simulink model "Microgrid_W"  (R2020a)
settings: Solver=ode15s  StartTime=0  StopTime=1440*1  MaxStep=1  RelTol=1e-3
libraries: simulink x4214, powerlib x685, simulink_extras x28, Microgrid_Library x18, powerlib_meascontrol x12
(part 44 of 48)

== system Microgrid_W/House 5 W2/Tv/D1 ==
  Add : Sum
  Clock : Clock
  Constant : Constant
  Constant1 : Constant  Value=0
  Gain : Gain  Gain=t
  Interval Test : simulink/Logic and Bit Operations/Interval Test  IntervalClosedRight=on  uplimit=TV_Off_1  IntervalClosedLeft=on  lowlimit=TV_On_1  OutDataTypeStr=boolean
  Interval Test1 : simulink/Logic and Bit Operations/Interval Test  IntervalClosedRight=on  uplimit=TV_Off_2  IntervalClosedLeft=on  lowlimit=TV_On_2  OutDataTypeStr=boolean
  Switch : Switch  Criteria=u2 > Threshold  Threshold=0.5
  Switch1 : Switch  Criteria=u2 > Threshold  Threshold=0.5
  Out1 : Outport  VectorParamsAs1DForOutWhenUnconnected=off
  wires:
  Clock/1 -> Gain/1
  Interval Test/1 -> Switch/2
  Switch/1 -> Add/1
  Interval Test1/1 -> Switch1/2
  Add/1 -> Out1/1
  Constant1/1 -> Switch/3, Switch1/3
  Constant/1 -> Switch/1, Switch1/1
  Switch1/1 -> Add/2
  Gain/1 -> Interval Test1/1, Interval Test/1

== system Microgrid_W/House 5 W2/Tv/D2 ==
  Add : Sum
  Clock : Clock
  Constant : Constant
  Constant1 : Constant  Value=0
  Gain : Gain  Gain=t
  Interval Test : simulink/Logic and Bit Operations/Interval Test  IntervalClosedRight=on  uplimit=TV_Off_1+86400  IntervalClosedLeft=on  lowlimit=TV_On_1+86400  OutDataTypeStr=boolean
  Interval Test1 : simulink/Logic and Bit Operations/Interval Test  IntervalClosedRight=on  uplimit=TV_Off_2+86400  IntervalClosedLeft=on  lowlimit=TV_On_2+86400  OutDataTypeStr=boolean
  Switch : Switch  Criteria=u2 > Threshold  Threshold=0.5
  Switch1 : Switch  Criteria=u2 > Threshold  Threshold=0.5
  Out1 : Outport  VectorParamsAs1DForOutWhenUnconnected=off
  wires:
  Clock/1 -> Gain/1
  Gain/1 -> Interval Test/1, Interval Test1/1
  Switch1/1 -> Add/2
  Constant/1 -> Switch1/1, Switch/1
  Constant1/1 -> Switch1/3, Switch/3
  Add/1 -> Out1/1
  Interval Test1/1 -> Switch1/2
  Switch/1 -> Add/1
  Interval Test/1 -> Switch/2

== system Microgrid_W/House 5 W2/Tv/D3 ==
  Add : Sum
  Clock : Clock
  Constant : Constant
  Constant1 : Constant  Value=0
  Gain : Gain  Gain=t
  Interval Test : simulink/Logic and Bit Operations/Interval Test  IntervalClosedRight=on  uplimit=TV_Off_1+86400*2  IntervalClosedLeft=on  lowlimit=TV_On_1+86400*2  OutDataTypeStr=boolean
  Interval Test1 : simulink/Logic and Bit Operations/Interval Test  IntervalClosedRight=on  uplimit=TV_Off_2+86400*2  IntervalClosedLeft=on  lowlimit=TV_On_2+86400*2  OutDataTypeStr=boolean
  Switch : Switch  Criteria=u2 > Threshold  Threshold=0.5
  Switch1 : Switch  Criteria=u2 > Threshold  Threshold=0.5
  Out1 : Outport  VectorParamsAs1DForOutWhenUnconnected=off
  wires:
  Clock/1 -> Gain/1
  Interval Test/1 -> Switch/2
  Switch/1 -> Add/1
  Interval Test1/1 -> Switch1/2
  Add/1 -> Out1/1
  Constant1/1 -> Switch/3, Switch1/3
  Constant/1 -> Switch/1, Switch1/1
  Switch1/1 -> Add/2
  Gain/1 -> Interval Test1/1, Interval Test/1

== system Microgrid_W/House 5 W2/Tv/D4 ==
  Add : Sum
  Clock : Clock
  Constant : Constant
  Constant1 : Constant  Value=0
  Gain : Gain  Gain=t
  Interval Test : simulink/Logic and Bit Operations/Interval Test  IntervalClosedRight=on  uplimit=TV_Off_1+86400*3  IntervalClosedLeft=on  lowlimit=TV_On_1+86400*3  OutDataTypeStr=boolean
  Interval Test1 : simulink/Logic and Bit Operations/Interval Test  IntervalClosedRight=on  uplimit=TV_Off_2+86400*3  IntervalClosedLeft=on  lowlimit=TV_On_2+86400*3  OutDataTypeStr=boolean
  Switch : Switch  Criteria=u2 > Threshold  Threshold=0.5
  Switch1 : Switch  Criteria=u2 > Threshold  Threshold=0.5
  Out1 : Outport  VectorParamsAs1DForOutWhenUnconnected=off
  wires:
  Clock/1 -> Gain/1
  Gain/1 -> Interval Test/1, Interval Test1/1
  Switch1/1 -> Add/2
  Constant/1 -> Switch1/1, Switch/1
  Constant1/1 -> Switch1/3, Switch/3
  Add/1 -> Out1/1
  Interval Test1/1 -> Switch1/2
  Switch/1 -> Add/1
  Interval Test/1 -> Switch/2

== system Microgrid_W/House 5 W2/Tv/D5 ==
  Add : Sum
  Clock : Clock
  Constant : Constant
  Constant1 : Constant  Value=0
  Gain : Gain  Gain=t
  Interval Test : simulink/Logic and Bit Operations/Interval Test  IntervalClosedRight=on  uplimit=TV_Off_1+86400*4  IntervalClosedLeft=on  lowlimit=TV_On_1+86400*4  OutDataTypeStr=boolean
  Interval Test1 : simulink/Logic and Bit Operations/Interval Test  IntervalClosedRight=on  uplimit=TV_Off_2+86400*4  IntervalClosedLeft=on  lowlimit=TV_On_2+86400*4  OutDataTypeStr=boolean
  Switch : Switch  Criteria=u2 > Threshold  Threshold=0.5
  Switch1 : Switch  Criteria=u2 > Threshold  Threshold=0.5
  Out1 : Outport  VectorParamsAs1DForOutWhenUnconnected=off
  wires:
  Clock/1 -> Gain/1
  Interval Test/1 -> Switch/2
  Switch/1 -> Add/1
  Interval Test1/1 -> Switch1/2
  Add/1 -> Out1/1
  Constant1/1 -> Switch/3, Switch1/3
  Constant/1 -> Switch/1, Switch1/1
  Switch1/1 -> Add/2
  Gain/1 -> Interval Test1/1, Interval Test/1

== system Microgrid_W/House 5 W2/Tv/D6 ==
  Add : Sum
  Clock : Clock
  Constant : Constant
  Constant1 : Constant  Value=0
  Gain : Gain  Gain=t
  Interval Test : simulink/Logic and Bit Operations/Interval Test  IntervalClosedRight=on  uplimit=TV_Off_1+86400*5  IntervalClosedLeft=on  lowlimit=TV_On_1+86400*5  OutDataTypeStr=boolean
  Interval Test1 : simulink/Logic and Bit Operations/Interval Test  IntervalClosedRight=on  uplimit=TV_Off_2+86400*5  IntervalClosedLeft=on  lowlimit=TV_On_2+86400*5  OutDataTypeStr=boolean
  Switch : Switch  Criteria=u2 > Threshold  Threshold=0.5
  Switch1 : Switch  Criteria=u2 > Threshold  Threshold=0.5
  Out1 : Outport  VectorParamsAs1DForOutWhenUnconnected=off
  wires:
  Clock/1 -> Gain/1
  Gain/1 -> Interval Test/1, Interval Test1/1
  Switch1/1 -> Add/2
  Constant/1 -> Switch1/1, Switch/1
  Constant1/1 -> Switch1/3, Switch/3
  Add/1 -> Out1/1
  Interval Test1/1 -> Switch1/2
  Switch/1 -> Add/1
  Interval Test/1 -> Switch/2

== system Microgrid_W/House 5 W2/Tv/D7 ==
  Add : Sum
  Clock : Clock
  Constant : Constant
  Constant1 : Constant  Value=0
  Gain : Gain  Gain=t
  Interval Test : simulink/Logic and Bit Operations/Interval Test  IntervalClosedRight=on  uplimit=TV_Off_1+86400*6  IntervalClosedLeft=on  lowlimit=TV_On_1+86400*6  OutDataTypeStr=boolean
  Interval Test1 : simulink/Logic and Bit Operations/Interval Test  IntervalClosedRight=on  uplimit=TV_Off_2+86400*6  IntervalClosedLeft=on  lowlimit=TV_On_2+86400*6  OutDataTypeStr=boolean
  Switch : Switch  Criteria=u2 > Threshold  Threshold=0.5
  Switch1 : Switch  Criteria=u2 > Threshold  Threshold=0.5
  Out1 : Outport  VectorParamsAs1DForOutWhenUnconnected=off
  wires:
  Clock/1 -> Gain/1
  Interval Test/1 -> Switch/2
  Switch/1 -> Add/1
  Interval Test1/1 -> Switch1/2
  Add/1 -> Out1/1
  Constant1/1 -> Switch/3, Switch1/3
  Constant/1 -> Switch/1, Switch1/1
  Switch1/1 -> Add/2
  Gain/1 -> Interval Test1/1, Interval Test/1

== system Microgrid_W/House 5 W2/Water tank/Thermostat ==
  In1 : Inport
  Compare To Constant : simulink/Logic and Bit Operations/Compare To Constant  relop=>=  const=T_High_WH  OutDataTypeStr=boolean
  Compare To Constant1 : simulink/Logic and Bit Operations/Compare To Constant  relop=<=  const=T_Low_WH  OutDataTypeStr=boolean
  Constant : Constant  Value=0
  Constant1 : Constant
  S-R Flip-Flop : simulink_extras/Flip Flops/S-R Flip-Flop  initial_condition=0
  Switch : Switch  Criteria=u2 > Threshold  Threshold=0.5
  Out1 : Outport  VectorParamsAs1DForOutWhenUnconnected=off
  wires:
  Constant/1 -> Switch/3
  Constant1/1 -> Switch/1
  Switch/1 -> Out1/1
  S-R Flip-Flop/1 -> Switch/2
  Compare To Constant1/1 -> S-R Flip-Flop/1
  Compare To Constant/1 -> S-R Flip-Flop/2
  In1/1 -> Compare To Constant/1, Compare To Constant1/1

== system Microgrid_W/House 5 W3/Heater/D1 ==
  Clock : Clock
  Constant : Constant
  Constant1 : Constant  Value=0
  Gain : Gain  Gain=t
  Interval Test : simulink/Logic and Bit Operations/Interval Test  IntervalClosedRight=on  uplimit=Heater_Off_1  IntervalClosedLeft=on  lowlimit=Heater_On_1  OutDataTypeStr=boolean
  Switch : Switch  Criteria=u2 > Threshold  Threshold=0.5
  Out1 : Outport  VectorParamsAs1DForOutWhenUnconnected=off
  wires:
  Interval Test/1 -> Switch/2
  Switch/1 -> Out1/1
  Constant1/1 -> Switch/3
  Constant/1 -> Switch/1
  Gain/1 -> Interval Test/1
  Clock/1 -> Gain/1

== system Microgrid_W/House 5 W3/Heater/D2 ==
  Clock : Clock
  Constant : Constant
  Constant1 : Constant  Value=0
  Gain : Gain  Gain=t
  Interval Test : simulink/Logic and Bit Operations/Interval Test  IntervalClosedRight=on  uplimit=Heater_Off_1+86400  IntervalClosedLeft=on  lowlimit=Heater_On_1+86400  OutDataTypeStr=boolean
  Switch : Switch  Criteria=u2 > Threshold  Threshold=0.5
  Out1 : Outport  VectorParamsAs1DForOutWhenUnconnected=off
  wires:
  Constant/1 -> Switch/1
  Constant1/1 -> Switch/3
  Switch/1 -> Out1/1
  Interval Test/1 -> Switch/2
  Gain/1 -> Interval Test/1
  Clock/1 -> Gain/1

== system Microgrid_W/House 5 W3/Heater/D3 ==
  Clock : Clock
  Constant : Constant
  Constant1 : Constant  Value=0
  Gain : Gain  Gain=t
  Interval Test : simulink/Logic and Bit Operations/Interval Test  IntervalClosedRight=on  uplimit=Heater_Off_1+86400*2  IntervalClosedLeft=on  lowlimit=Heater_On_1+86400*2  OutDataTypeStr=boolean
  Switch : Switch  Criteria=u2 > Threshold  Threshold=0.5
  Out1 : Outport  VectorParamsAs1DForOutWhenUnconnected=off
  wires:
  Interval Test/1 -> Switch/2
  Switch/1 -> Out1/1
  Constant1/1 -> Switch/3
  Constant/1 -> Switch/1
  Gain/1 -> Interval Test/1
  Clock/1 -> Gain/1

== system Microgrid_W/House 5 W3/Heater/D4 ==
  Clock : Clock
  Constant : Constant
  Constant1 : Constant  Value=0
  Gain : Gain  Gain=t
  Interval Test : simulink/Logic and Bit Operations/Interval Test  IntervalClosedRight=on  uplimit=Heater_Off_1+86400*3  IntervalClosedLeft=on  lowlimit=Heater_On_1+86400*3  OutDataTypeStr=boolean
  Switch : Switch  Criteria=u2 > Threshold  Threshold=0.5
  Out1 : Outport  VectorParamsAs1DForOutWhenUnconnected=off
  wires:
  Constant/1 -> Switch/1
  Constant1/1 -> Switch/3
  Switch/1 -> Out1/1
  Interval Test/1 -> Switch/2
  Gain/1 -> Interval Test/1
  Clock/1 -> Gain/1

== system Microgrid_W/House 5 W3/Heater/D5 ==
  Clock : Clock
  Constant : Constant
  Constant1 : Constant  Value=0
  Gain : Gain  Gain=t
  Interval Test : simulink/Logic and Bit Operations/Interval Test  IntervalClosedRight=on  uplimit=Heater_Off_1+86400*4  IntervalClosedLeft=on  lowlimit=Heater_On_1+86400*4  OutDataTypeStr=boolean
  Switch : Switch  Criteria=u2 > Threshold  Threshold=0.5
  Out1 : Outport  VectorParamsAs1DForOutWhenUnconnected=off
  wires:
  Interval Test/1 -> Switch/2
  Switch/1 -> Out1/1
  Constant1/1 -> Switch/3
  Constant/1 -> Switch/1
  Gain/1 -> Interval Test/1
  Clock/1 -> Gain/1

== system Microgrid_W/House 5 W3/Heater/D6 ==
  Clock : Clock
  Constant : Constant
  Constant1 : Constant  Value=0
  Gain : Gain  Gain=t
  Interval Test : simulink/Logic and Bit Operations/Interval Test  IntervalClosedRight=on  uplimit=Heater_Off_1+86400*5  IntervalClosedLeft=on  lowlimit=Heater_On_1+86400*5  OutDataTypeStr=boolean
  Switch : Switch  Criteria=u2 > Threshold  Threshold=0.5
  Out1 : Outport  VectorParamsAs1DForOutWhenUnconnected=off
  wires:
  Gain/1 -> Interval Test/1
  Constant/1 -> Switch/1
  Constant1/1 -> Switch/3
  Switch/1 -> Out1/1
  Interval Test/1 -> Switch/2
  Clock/1 -> Gain/1

== system Microgrid_W/House 5 W3/Heater/D7 ==
  Clock : Clock
  Constant : Constant
  Constant1 : Constant  Value=0
  Gain : Gain  Gain=t
  Interval Test : simulink/Logic and Bit Operations/Interval Test  IntervalClosedRight=on  uplimit=Heater_Off_1+86400*6  IntervalClosedLeft=on  lowlimit=Heater_On_1+86400*6  OutDataTypeStr=boolean
  Switch : Switch  Criteria=u2 > Threshold  Threshold=0.5
  Out1 : Outport  VectorParamsAs1DForOutWhenUnconnected=off
  wires:
  Interval Test/1 -> Switch/2
  Switch/1 -> Out1/1
  Constant1/1 -> Switch/3
  Constant/1 -> Switch/1
  Gain/1 -> Interval Test/1
  Clock/1 -> Gain/1

== system Microgrid_W/House 5 W3/Kettle/D1 ==
  Add : Sum  Inputs=+++
  Clock : Clock
  Compare To Zero : simulink/Logic and Bit Operations/Compare To Zero  relop=>  OutDataTypeStr=boolean
  Compare To Zero1 : simulink/Logic and Bit Operations/Compare To Zero  relop=>  OutDataTypeStr=boolean
  Compare To Zero2 : simulink/Logic and Bit Operations/Compare To Zero  relop=>  OutDataTypeStr=boolean
  Constant : Constant
  Constant{1..2,5,8} (4 alike) : Constant  Value=0
  Constant3 : Constant  Value=Jug_On_1
  Constant4 : Constant
  Constant6 : Constant  Value=Jug_On_2
  Constant7 : Constant
  Constant9 : Constant  Value=Jug_On_3
  Gain : Gain  Gain=t
  Interval Test : simulink/Logic and Bit Operations/Interval Test  IntervalClosedRight=on  uplimit=Jug_On_1+180  IntervalClosedLeft=on  lowlimit=Jug_On_1  OutDataTypeStr=boolean
  Interval Test1 : simulink/Logic and Bit Operations/Interval Test  IntervalClosedRight=on  uplimit=Jug_On_2+180  IntervalClosedLeft=on  lowlimit=Jug_On_2  OutDataTypeStr=boolean
  Interval Test2 : simulink/Logic and Bit Operations/Interval Test  IntervalClosedRight=on  uplimit=Jug_On_3+180  IntervalClosedLeft=on  lowlimit=Jug_On_3  OutDataTypeStr=boolean
  Switch{,1..5} (6 alike) : Switch  Criteria=u2 > Threshold  Threshold=0.5
  Out1 : Outport  VectorParamsAs1DForOutWhenUnconnected=off
  wires:
  Interval Test/1 -> Switch/2
  Constant1/1 -> Switch3/3, Switch2/3, Switch/3
  Gain/1 -> Interval Test2/1, Interval Test1/1, Interval Test/1
  Constant3/1 -> Compare To Zero/1
  Constant/1 -> Switch1/1
  Constant2/1 -> Switch1/3
  Compare To Zero/1 -> Switch1/2
  Switch1/1 -> Switch/1
  Interval Test1/1 -> Switch2/2
  Interval Test2/1 -> Switch3/2
  Constant6/1 -> Compare To Zero1/1
  Constant4/1 -> Switch4/1
  Constant5/1 -> Switch4/3
  Compare To Zero1/1 -> Switch4/2
  Constant9/1 -> Compare To Zero2/1
  Constant7/1 -> Switch5/1
  Constant8/1 -> Switch5/3
  Compare To Zero2/1 -> Switch5/2
  Switch4/1 -> Switch2/1
  Switch5/1 -> Switch3/1
  Switch/1 -> Add/1
  Switch2/1 -> Add/2
  Switch3/1 -> Add/3
  Add/1 -> Out1/1
  Clock/1 -> Gain/1

== system Microgrid_W/House 5 W3/Kettle/D2 ==
  Add : Sum  Inputs=+++
  Clock : Clock
  Compare To Zero : simulink/Logic and Bit Operations/Compare To Zero  relop=>  OutDataTypeStr=boolean
  Compare To Zero1 : simulink/Logic and Bit Operations/Compare To Zero  relop=>  OutDataTypeStr=boolean
  Compare To Zero2 : simulink/Logic and Bit Operations/Compare To Zero  relop=>  OutDataTypeStr=boolean
  Constant : Constant
  Constant{1..2,5,8} (4 alike) : Constant  Value=0
  Constant3 : Constant  Value=Jug_On_1
  Constant4 : Constant
  Constant6 : Constant  Value=Jug_On_2
  Constant7 : Constant
  Constant9 : Constant  Value=Jug_On_3
  Gain : Gain  Gain=t
  Interval Test : simulink/Logic and Bit Operations/Interval Test  IntervalClosedRight=on  uplimit=Jug_On_1+180+86400  IntervalClosedLeft=on  lowlimit=Jug_On_1+86400  OutDataTypeStr=boolean
  Interval Test1 : simulink/Logic and Bit Operations/Interval Test  IntervalClosedRight=on  uplimit=Jug_On_2+180+86400  IntervalClosedLeft=on  lowlimit=Jug_On_2+86400  OutDataTypeStr=boolean
  Interval Test2 : simulink/Logic and Bit Operations/Interval Test  IntervalClosedRight=on  uplimit=Jug_On_3+180+86400  IntervalClosedLeft=on  lowlimit=Jug_On_3+86400  OutDataTypeStr=boolean
  Switch{,1..5} (6 alike) : Switch  Criteria=u2 > Threshold  Threshold=0.5
  Out1 : Outport  VectorParamsAs1DForOutWhenUnconnected=off
  wires:
  Add/1 -> Out1/1
  Switch3/1 -> Add/3
  Switch2/1 -> Add/2
  Switch/1 -> Add/1
  Switch5/1 -> Switch3/1
  Switch4/1 -> Switch2/1
  Compare To Zero2/1 -> Switch5/2
  Constant8/1 -> Switch5/3
  Constant7/1 -> Switch5/1
  Constant9/1 -> Compare To Zero2/1
  Compare To Zero1/1 -> Switch4/2
  Constant5/1 -> Switch4/3
  Constant4/1 -> Switch4/1
  Constant6/1 -> Compare To Zero1/1
  Interval Test2/1 -> Switch3/2
  Interval Test1/1 -> Switch2/2
  Switch1/1 -> Switch/1
  Compare To Zero/1 -> Switch1/2
  Constant2/1 -> Switch1/3
  Constant/1 -> Switch1/1
  Constant3/1 -> Compare To Zero/1
  Gain/1 -> Interval Test/1, Interval Test1/1, Interval Test2/1
  Constant1/1 -> Switch/3, Switch2/3, Switch3/3
  Interval Test/1 -> Switch/2
  Clock/1 -> Gain/1

== system Microgrid_W/House 5 W3/Kettle/D3 ==
  Add : Sum  Inputs=+++
  Clock : Clock
  Compare To Zero : simulink/Logic and Bit Operations/Compare To Zero  relop=>  OutDataTypeStr=boolean
  Compare To Zero1 : simulink/Logic and Bit Operations/Compare To Zero  relop=>  OutDataTypeStr=boolean
  Compare To Zero2 : simulink/Logic and Bit Operations/Compare To Zero  relop=>  OutDataTypeStr=boolean
  Constant : Constant
  Constant{1..2,5,8} (4 alike) : Constant  Value=0
  Constant3 : Constant  Value=Jug_On_1
  Constant4 : Constant
  Constant6 : Constant  Value=Jug_On_2
  Constant7 : Constant
  Constant9 : Constant  Value=Jug_On_3
  Gain : Gain  Gain=t
  Interval Test : simulink/Logic and Bit Operations/Interval Test  IntervalClosedRight=on  uplimit=Jug_On_1+180+86400*2  IntervalClosedLeft=on  lowlimit=Jug_On_1+86400*2  OutDataTypeStr=boolean
  Interval Test1 : simulink/Logic and Bit Operations/Interval Test  IntervalClosedRight=on  uplimit=Jug_On_2+180+86400*2  IntervalClosedLeft=on  lowlimit=Jug_On_2+86400*2  OutDataTypeStr=boolean
  Interval Test2 : simulink/Logic and Bit Operations/Interval Test  IntervalClosedRight=on  uplimit=Jug_On_3+180+86400*2  IntervalClosedLeft=on  lowlimit=Jug_On_3+86400*2  OutDataTypeStr=boolean
  Switch{,1..5} (6 alike) : Switch  Criteria=u2 > Threshold  Threshold=0.5
  Out1 : Outport  VectorParamsAs1DForOutWhenUnconnected=off
  wires:
  Interval Test/1 -> Switch/2
  Constant1/1 -> Switch3/3, Switch2/3, Switch/3
  Gain/1 -> Interval Test2/1, Interval Test1/1, Interval Test/1
  Constant3/1 -> Compare To Zero/1
  Constant/1 -> Switch1/1
  Constant2/1 -> Switch1/3
  Compare To Zero/1 -> Switch1/2
  Switch1/1 -> Switch/1
  Interval Test1/1 -> Switch2/2
  Interval Test2/1 -> Switch3/2
  Constant6/1 -> Compare To Zero1/1
  Constant4/1 -> Switch4/1
  Constant5/1 -> Switch4/3
  Compare To Zero1/1 -> Switch4/2
  Constant9/1 -> Compare To Zero2/1
  Constant7/1 -> Switch5/1
  Constant8/1 -> Switch5/3
  Compare To Zero2/1 -> Switch5/2
  Switch4/1 -> Switch2/1
  Switch5/1 -> Switch3/1
  Switch/1 -> Add/1
  Switch2/1 -> Add/2
  Switch3/1 -> Add/3
  Add/1 -> Out1/1
  Clock/1 -> Gain/1

== system Microgrid_W/House 5 W3/Kettle/D4 ==
  Add : Sum  Inputs=+++
  Clock : Clock
  Compare To Zero : simulink/Logic and Bit Operations/Compare To Zero  relop=>  OutDataTypeStr=boolean
  Compare To Zero1 : simulink/Logic and Bit Operations/Compare To Zero  relop=>  OutDataTypeStr=boolean
  Compare To Zero2 : simulink/Logic and Bit Operations/Compare To Zero  relop=>  OutDataTypeStr=boolean
  Constant : Constant
  Constant{1..2,5,8} (4 alike) : Constant  Value=0
  Constant3 : Constant  Value=Jug_On_1
  Constant4 : Constant
  Constant6 : Constant  Value=Jug_On_2
  Constant7 : Constant
  Constant9 : Constant  Value=Jug_On_3
  Gain : Gain  Gain=t
  Interval Test : simulink/Logic and Bit Operations/Interval Test  IntervalClosedRight=on  uplimit=Jug_On_1+180+86400*3  IntervalClosedLeft=on  lowlimit=Jug_On_1+86400*3  OutDataTypeStr=boolean
  Interval Test1 : simulink/Logic and Bit Operations/Interval Test  IntervalClosedRight=on  uplimit=Jug_On_2+180+86400*3  IntervalClosedLeft=on  lowlimit=Jug_On_2+86400*3  OutDataTypeStr=boolean
  Interval Test2 : simulink/Logic and Bit Operations/Interval Test  IntervalClosedRight=on  uplimit=Jug_On_3+180+86400*3  IntervalClosedLeft=on  lowlimit=Jug_On_3+86400*3  OutDataTypeStr=boolean
  Switch{,1..5} (6 alike) : Switch  Criteria=u2 > Threshold  Threshold=0.5
  Out1 : Outport  VectorParamsAs1DForOutWhenUnconnected=off
  wires:
  Add/1 -> Out1/1
  Switch3/1 -> Add/3
  Switch2/1 -> Add/2
  Switch/1 -> Add/1
  Switch5/1 -> Switch3/1
  Switch4/1 -> Switch2/1
  Compare To Zero2/1 -> Switch5/2
  Constant8/1 -> Switch5/3
  Constant7/1 -> Switch5/1
  Constant9/1 -> Compare To Zero2/1
  Compare To Zero1/1 -> Switch4/2
  Constant5/1 -> Switch4/3
  Constant4/1 -> Switch4/1
  Constant6/1 -> Compare To Zero1/1
  Interval Test2/1 -> Switch3/2
  Interval Test1/1 -> Switch2/2
  Switch1/1 -> Switch/1
  Compare To Zero/1 -> Switch1/2
  Constant2/1 -> Switch1/3
  Constant/1 -> Switch1/1
  Constant3/1 -> Compare To Zero/1
  Gain/1 -> Interval Test/1, Interval Test1/1, Interval Test2/1
  Constant1/1 -> Switch/3, Switch2/3, Switch3/3
  Interval Test/1 -> Switch/2
  Clock/1 -> Gain/1

== system Microgrid_W/House 5 W3/Kettle/D5 ==
  Add : Sum  Inputs=+++
  Clock : Clock
  Compare To Zero : simulink/Logic and Bit Operations/Compare To Zero  relop=>  OutDataTypeStr=boolean
  Compare To Zero1 : simulink/Logic and Bit Operations/Compare To Zero  relop=>  OutDataTypeStr=boolean
  Compare To Zero2 : simulink/Logic and Bit Operations/Compare To Zero  relop=>  OutDataTypeStr=boolean
  Constant : Constant
  Constant{1..2,5,8} (4 alike) : Constant  Value=0
  Constant3 : Constant  Value=Jug_On_1
  Constant4 : Constant
  Constant6 : Constant  Value=Jug_On_2
  Constant7 : Constant
  Constant9 : Constant  Value=Jug_On_3
  Gain : Gain  Gain=t
  Interval Test : simulink/Logic and Bit Operations/Interval Test  IntervalClosedRight=on  uplimit=Jug_On_1+180+86400*4  IntervalClosedLeft=on  lowlimit=Jug_On_1+86400*4  OutDataTypeStr=boolean
  Interval Test1 : simulink/Logic and Bit Operations/Interval Test  IntervalClosedRight=on  uplimit=Jug_On_2+180+86400*4  IntervalClosedLeft=on  lowlimit=Jug_On_2+86400*4  OutDataTypeStr=boolean
  Interval Test2 : simulink/Logic and Bit Operations/Interval Test  IntervalClosedRight=on  uplimit=Jug_On_3+180+86400*4  IntervalClosedLeft=on  lowlimit=Jug_On_3+86400*4  OutDataTypeStr=boolean
  Switch{,1..5} (6 alike) : Switch  Criteria=u2 > Threshold  Threshold=0.5
  Out1 : Outport  VectorParamsAs1DForOutWhenUnconnected=off
  wires:
  Interval Test/1 -> Switch/2
  Constant1/1 -> Switch3/3, Switch2/3, Switch/3
  Gain/1 -> Interval Test2/1, Interval Test1/1, Interval Test/1
  Constant3/1 -> Compare To Zero/1
  Constant/1 -> Switch1/1
  Constant2/1 -> Switch1/3
  Compare To Zero/1 -> Switch1/2
  Switch1/1 -> Switch/1
  Interval Test1/1 -> Switch2/2
  Interval Test2/1 -> Switch3/2
  Constant6/1 -> Compare To Zero1/1
  Constant4/1 -> Switch4/1
  Constant5/1 -> Switch4/3
  Compare To Zero1/1 -> Switch4/2
  Constant9/1 -> Compare To Zero2/1
  Constant7/1 -> Switch5/1
  Constant8/1 -> Switch5/3
  Compare To Zero2/1 -> Switch5/2
  Switch4/1 -> Switch2/1
  Switch5/1 -> Switch3/1
  Switch/1 -> Add/1
  Switch2/1 -> Add/2
  Switch3/1 -> Add/3
  Add/1 -> Out1/1
  Clock/1 -> Gain/1

== system Microgrid_W/House 5 W3/Kettle/D6 ==
  Add : Sum  Inputs=+++
  Clock : Clock
  Compare To Zero : simulink/Logic and Bit Operations/Compare To Zero  relop=>  OutDataTypeStr=boolean
  Compare To Zero1 : simulink/Logic and Bit Operations/Compare To Zero  relop=>  OutDataTypeStr=boolean
  Compare To Zero2 : simulink/Logic and Bit Operations/Compare To Zero  relop=>  OutDataTypeStr=boolean
  Constant : Constant
  Constant{1..2,5,8} (4 alike) : Constant  Value=0
  Constant3 : Constant  Value=Jug_On_1
  Constant4 : Constant
  Constant6 : Constant  Value=Jug_On_2
  Constant7 : Constant
  Constant9 : Constant  Value=Jug_On_3
  Gain : Gain  Gain=t
  Interval Test : simulink/Logic and Bit Operations/Interval Test  IntervalClosedRight=on  uplimit=Jug_On_1+180+86400*5  IntervalClosedLeft=on  lowlimit=Jug_On_1+86400*5  OutDataTypeStr=boolean
  Interval Test1 : simulink/Logic and Bit Operations/Interval Test  IntervalClosedRight=on  uplimit=Jug_On_2+180+86400*5  IntervalClosedLeft=on  lowlimit=Jug_On_2+86400*5  OutDataTypeStr=boolean
  Interval Test2 : simulink/Logic and Bit Operations/Interval Test  IntervalClosedRight=on  uplimit=Jug_On_3+180+86400*5  IntervalClosedLeft=on  lowlimit=Jug_On_3+86400*5  OutDataTypeStr=boolean
  Switch{,1..5} (6 alike) : Switch  Criteria=u2 > Threshold  Threshold=0.5
  Out1 : Outport  VectorParamsAs1DForOutWhenUnconnected=off
  wires:
  Add/1 -> Out1/1
  Switch3/1 -> Add/3
  Switch2/1 -> Add/2
  Switch/1 -> Add/1
  Switch5/1 -> Switch3/1
  Switch4/1 -> Switch2/1
  Compare To Zero2/1 -> Switch5/2
  Constant8/1 -> Switch5/3
  Constant7/1 -> Switch5/1
  Constant9/1 -> Compare To Zero2/1
  Compare To Zero1/1 -> Switch4/2
  Constant5/1 -> Switch4/3
  Constant4/1 -> Switch4/1
  Constant6/1 -> Compare To Zero1/1
  Interval Test2/1 -> Switch3/2
  Interval Test1/1 -> Switch2/2
  Switch1/1 -> Switch/1
  Compare To Zero/1 -> Switch1/2
  Constant2/1 -> Switch1/3
  Constant/1 -> Switch1/1
  Constant3/1 -> Compare To Zero/1
  Gain/1 -> Interval Test/1, Interval Test1/1, Interval Test2/1
  Constant1/1 -> Switch/3, Switch2/3, Switch3/3
  Interval Test/1 -> Switch/2
  Clock/1 -> Gain/1

== system Microgrid_W/House 5 W3/Kettle/D7 ==
  Add : Sum  Inputs=+++
  Clock : Clock
  Compare To Zero : simulink/Logic and Bit Operations/Compare To Zero  relop=>  OutDataTypeStr=boolean
  Compare To Zero1 : simulink/Logic and Bit Operations/Compare To Zero  relop=>  OutDataTypeStr=boolean
  Compare To Zero2 : simulink/Logic and Bit Operations/Compare To Zero  relop=>  OutDataTypeStr=boolean
  Constant : Constant
  Constant{1..2,5,8} (4 alike) : Constant  Value=0
  Constant3 : Constant  Value=Jug_On_1
  Constant4 : Constant
  Constant6 : Constant  Value=Jug_On_2
  Constant7 : Constant
  Constant9 : Constant  Value=Jug_On_3
  Gain : Gain  Gain=t
  Interval Test : simulink/Logic and Bit Operations/Interval Test  IntervalClosedRight=on  uplimit=Jug_On_1+180+86400*6  IntervalClosedLeft=on  lowlimit=Jug_On_1+86400*6  OutDataTypeStr=boolean
  Interval Test1 : simulink/Logic and Bit Operations/Interval Test  IntervalClosedRight=on  uplimit=Jug_On_2+180+86400*6  IntervalClosedLeft=on  lowlimit=Jug_On_2+86400*6  OutDataTypeStr=boolean
  Interval Test2 : simulink/Logic and Bit Operations/Interval Test  IntervalClosedRight=on  uplimit=Jug_On_3+180+86400*6  IntervalClosedLeft=on  lowlimit=Jug_On_3+86400*6  OutDataTypeStr=boolean
  Switch{,1..5} (6 alike) : Switch  Criteria=u2 > Threshold  Threshold=0.5
  Out1 : Outport  VectorParamsAs1DForOutWhenUnconnected=off
  wires:
  Interval Test/1 -> Switch/2
  Constant1/1 -> Switch3/3, Switch2/3, Switch/3
  Gain/1 -> Interval Test2/1, Interval Test1/1, Interval Test/1
  Constant3/1 -> Compare To Zero/1
  Constant/1 -> Switch1/1
  Constant2/1 -> Switch1/3
  Compare To Zero/1 -> Switch1/2
  Switch1/1 -> Switch/1
  Interval Test1/1 -> Switch2/2
  Interval Test2/1 -> Switch3/2
  Constant6/1 -> Compare To Zero1/1
  Constant4/1 -> Switch4/1
  Constant5/1 -> Switch4/3
  Compare To Zero1/1 -> Switch4/2
  Constant9/1 -> Compare To Zero2/1
  Constant7/1 -> Switch5/1
  Constant8/1 -> Switch5/3
  Compare To Zero2/1 -> Switch5/2
  Switch4/1 -> Switch2/1
  Switch5/1 -> Switch3/1
  Switch/1 -> Add/1
  Switch2/1 -> Add/2
  Switch3/1 -> Add/3
  Add/1 -> Out1/1
  Clock/1 -> Gain/1

== system Microgrid_W/House 5 W3/Lamp 1/D1 ==
  Add : Sum
  Clock : Clock
  Constant : Constant
  Constant1 : Constant  Value=0
  Gain : Gain  Gain=t
  Interval Test : simulink/Logic and Bit Operations/Interval Test  IntervalClosedRight=on  uplimit=L1_Off_1  IntervalClosedLeft=on  lowlimit=L1_On_1  OutDataTypeStr=boolean
  Interval Test1 : simulink/Logic and Bit Operations/Interval Test  IntervalClosedRight=on  uplimit=L1_Off_2  IntervalClosedLeft=on  lowlimit=L1_On_2  OutDataTypeStr=boolean
  Switch : Switch  Criteria=u2 > Threshold  Threshold=0.5
  Switch1 : Switch  Criteria=u2 > Threshold  Threshold=0.5
  Out1 : Outport  VectorParamsAs1DForOutWhenUnconnected=off
  wires:
  Gain/1 -> Interval Test/1, Interval Test1/1
  Switch1/1 -> Add/2
  Constant/1 -> Switch1/1, Switch/1
  Constant1/1 -> Switch1/3, Switch/3
  Add/1 -> Out1/1
  Interval Test1/1 -> Switch1/2
  Switch/1 -> Add/1
  Interval Test/1 -> Switch/2
  Clock/1 -> Gain/1

== system Microgrid_W/House 5 W3/Lamp 1/D2 ==
  Add : Sum
  Clock : Clock
  Constant : Constant
  Constant1 : Constant  Value=0
  Gain : Gain  Gain=t
  Interval Test : simulink/Logic and Bit Operations/Interval Test  IntervalClosedRight=on  uplimit=L1_Off_1+86400  IntervalClosedLeft=on  lowlimit=L1_On_1+86400  OutDataTypeStr=boolean
  Interval Test1 : simulink/Logic and Bit Operations/Interval Test  IntervalClosedRight=on  uplimit=L1_Off_2+86400  IntervalClosedLeft=on  lowlimit=L1_On_2+86400  OutDataTypeStr=boolean
  Switch : Switch  Criteria=u2 > Threshold  Threshold=0.5
  Switch1 : Switch  Criteria=u2 > Threshold  Threshold=0.5
  Out1 : Outport  VectorParamsAs1DForOutWhenUnconnected=off
  wires:
  Interval Test/1 -> Switch/2
  Switch/1 -> Add/1
  Interval Test1/1 -> Switch1/2
  Add/1 -> Out1/1
  Constant1/1 -> Switch/3, Switch1/3
  Constant/1 -> Switch/1, Switch1/1
  Switch1/1 -> Add/2
  Gain/1 -> Interval Test1/1, Interval Test/1
  Clock/1 -> Gain/1

== system Microgrid_W/House 5 W3/Lamp 1/D3 ==
  Add : Sum
  Clock : Clock
  Constant : Constant
  Constant1 : Constant  Value=0
  Gain : Gain  Gain=t
  Interval Test : simulink/Logic and Bit Operations/Interval Test  IntervalClosedRight=on  uplimit=L1_Off_1+86400*2  IntervalClosedLeft=on  lowlimit=L1_On_1+86400*2  OutDataTypeStr=boolean
  Interval Test1 : simulink/Logic and Bit Operations/Interval Test  IntervalClosedRight=on  uplimit=L1_Off_2+86400*2  IntervalClosedLeft=on  lowlimit=L1_On_2+86400*2  OutDataTypeStr=boolean
  Switch : Switch  Criteria=u2 > Threshold  Threshold=0.5
  Switch1 : Switch  Criteria=u2 > Threshold  Threshold=0.5
  Out1 : Outport  VectorParamsAs1DForOutWhenUnconnected=off
  wires:
  Gain/1 -> Interval Test/1, Interval Test1/1
  Switch1/1 -> Add/2
  Constant/1 -> Switch1/1, Switch/1
  Constant1/1 -> Switch1/3, Switch/3
  Add/1 -> Out1/1
  Interval Test1/1 -> Switch1/2
  Switch/1 -> Add/1
  Interval Test/1 -> Switch/2
  Clock/1 -> Gain/1

== system Microgrid_W/House 5 W3/Lamp 1/D4 ==
  Add : Sum
  Clock : Clock
  Constant : Constant
  Constant1 : Constant  Value=0
  Gain : Gain  Gain=t
  Interval Test : simulink/Logic and Bit Operations/Interval Test  IntervalClosedRight=on  uplimit=L1_Off_1+86400*3  IntervalClosedLeft=on  lowlimit=L1_On_1+86400*3  OutDataTypeStr=boolean
  Interval Test1 : simulink/Logic and Bit Operations/Interval Test  IntervalClosedRight=on  uplimit=L1_Off_2+86400*3  IntervalClosedLeft=on  lowlimit=L1_On_2+86400*3  OutDataTypeStr=boolean
  Switch : Switch  Criteria=u2 > Threshold  Threshold=0.5
  Switch1 : Switch  Criteria=u2 > Threshold  Threshold=0.5
  Out1 : Outport  VectorParamsAs1DForOutWhenUnconnected=off
  wires:
  Interval Test/1 -> Switch/2
  Switch/1 -> Add/1
  Interval Test1/1 -> Switch1/2
  Add/1 -> Out1/1
  Constant1/1 -> Switch/3, Switch1/3
  Constant/1 -> Switch/1, Switch1/1
  Switch1/1 -> Add/2
  ? -> Interval Test1/1, Interval Test/1
  Clock/1 -> Gain/1

== system Microgrid_W/House 5 W3/Lamp 1/D5 ==
  Add : Sum
  Clock : Clock
  Constant : Constant
  Constant1 : Constant  Value=0
  Gain : Gain  Gain=t
  Interval Test : simulink/Logic and Bit Operations/Interval Test  IntervalClosedRight=on  uplimit=L1_Off_1+86400*4  IntervalClosedLeft=on  lowlimit=L1_On_1+86400*4  OutDataTypeStr=boolean
  Interval Test1 : simulink/Logic and Bit Operations/Interval Test  IntervalClosedRight=on  uplimit=L1_Off_2+86400*4  IntervalClosedLeft=on  lowlimit=L1_On_2+86400*4  OutDataTypeStr=boolean
  Switch : Switch  Criteria=u2 > Threshold  Threshold=0.5
  Switch1 : Switch  Criteria=u2 > Threshold  Threshold=0.5
  Out1 : Outport  VectorParamsAs1DForOutWhenUnconnected=off
  wires:
  Gain/1 -> Interval Test/1, Interval Test1/1
  Switch1/1 -> Add/2
  Constant/1 -> Switch1/1, Switch/1
  Constant1/1 -> Switch1/3, Switch/3
  Add/1 -> Out1/1
  Interval Test1/1 -> Switch1/2
  Switch/1 -> Add/1
  Interval Test/1 -> Switch/2
  Clock/1 -> Gain/1

== system Microgrid_W/House 5 W3/Lamp 1/D6 ==
  Add : Sum
  Clock : Clock
  Constant : Constant
  Constant1 : Constant  Value=0
  Gain : Gain  Gain=t
  Interval Test : simulink/Logic and Bit Operations/Interval Test  IntervalClosedRight=on  uplimit=L1_Off_1+86400*5  IntervalClosedLeft=on  lowlimit=L1_On_1+86400*5  OutDataTypeStr=boolean
  Interval Test1 : simulink/Logic and Bit Operations/Interval Test  IntervalClosedRight=on  uplimit=L1_Off_2+86400*5  IntervalClosedLeft=on  lowlimit=L1_On_2+86400*5  OutDataTypeStr=boolean
  Switch : Switch  Criteria=u2 > Threshold  Threshold=0.5
  Switch1 : Switch  Criteria=u2 > Threshold  Threshold=0.5
  Out1 : Outport  VectorParamsAs1DForOutWhenUnconnected=off
  wires:
  Interval Test/1 -> Switch/2
  Switch/1 -> Add/1
  Interval Test1/1 -> Switch1/2
  Add/1 -> Out1/1
  Constant1/1 -> Switch/3, Switch1/3
  Constant/1 -> Switch/1, Switch1/1
  Switch1/1 -> Add/2
  Gain/1 -> Interval Test1/1, Interval Test/1
  Clock/1 -> Gain/1

== system Microgrid_W/House 5 W3/Lamp 1/D7 ==
  Add : Sum
  Clock : Clock
  Constant : Constant
  Constant1 : Constant  Value=0
  Gain : Gain  Gain=t
  Interval Test : simulink/Logic and Bit Operations/Interval Test  IntervalClosedRight=on  uplimit=L1_Off_1+86400*6  IntervalClosedLeft=on  lowlimit=L1_On_1+86400*6  OutDataTypeStr=boolean
  Interval Test1 : simulink/Logic and Bit Operations/Interval Test  IntervalClosedRight=on  uplimit=L1_Off_2+86400*6  IntervalClosedLeft=on  lowlimit=L1_On_2+86400*6  OutDataTypeStr=boolean
  Switch : Switch  Criteria=u2 > Threshold  Threshold=0.5
  Switch1 : Switch  Criteria=u2 > Threshold  Threshold=0.5
  Out1 : Outport  VectorParamsAs1DForOutWhenUnconnected=off
  wires:
  Gain/1 -> Interval Test/1, Interval Test1/1
  Switch1/1 -> Add/2
  Constant/1 -> Switch1/1, Switch/1
  Constant1/1 -> Switch1/3, Switch/3
  Add/1 -> Out1/1
  Interval Test1/1 -> Switch1/2
  Switch/1 -> Add/1
  Interval Test/1 -> Switch/2
  Clock/1 -> Gain/1

== system Microgrid_W/House 5 W3/Lamp 2/D1 ==
  Add : Sum
  Clock : Clock
  Constant : Constant
  Constant1 : Constant  Value=0
  Gain : Gain  Gain=t
  Interval Test : simulink/Logic and Bit Operations/Interval Test  IntervalClosedRight=on  uplimit=L2_Off_1  IntervalClosedLeft=on  lowlimit=L2_On_1  OutDataTypeStr=boolean
  Interval Test1 : simulink/Logic and Bit Operations/Interval Test  IntervalClosedRight=on  uplimit=L2_Off_2  IntervalClosedLeft=on  lowlimit=L2_On_2  OutDataTypeStr=boolean
  Switch : Switch  Criteria=u2 > Threshold  Threshold=0.5
  Switch1 : Switch  Criteria=u2 > Threshold  Threshold=0.5
  Out1 : Outport  VectorParamsAs1DForOutWhenUnconnected=off
  wires:
  Interval Test/1 -> Switch/2
  Switch/1 -> Add/1
  Interval Test1/1 -> Switch1/2
  Add/1 -> Out1/1
  Constant1/1 -> Switch/3, Switch1/3
  Constant/1 -> Switch/1, Switch1/1
  Switch1/1 -> Add/2
  Gain/1 -> Interval Test1/1, Interval Test/1
  Clock/1 -> Gain/1

== system Microgrid_W/House 5 W3/Lamp 2/D2 ==
  Add : Sum
  Clock : Clock
  Constant : Constant
  Constant1 : Constant  Value=0
  Gain : Gain  Gain=t
  Interval Test : simulink/Logic and Bit Operations/Interval Test  IntervalClosedRight=on  uplimit=L2_Off_1+86400  IntervalClosedLeft=on  lowlimit=L2_On_1+86400  OutDataTypeStr=boolean
  Interval Test1 : simulink/Logic and Bit Operations/Interval Test  IntervalClosedRight=on  uplimit=L2_Off_2+86400  IntervalClosedLeft=on  lowlimit=L2_On_2+86400  OutDataTypeStr=boolean
  Switch : Switch  Criteria=u2 > Threshold  Threshold=0.5
  Switch1 : Switch  Criteria=u2 > Threshold  Threshold=0.5
  Out1 : Outport  VectorParamsAs1DForOutWhenUnconnected=off
  wires:
  Gain/1 -> Interval Test/1, Interval Test1/1
  Switch1/1 -> Add/2
  Constant/1 -> Switch1/1, Switch/1
  Constant1/1 -> Switch1/3, Switch/3
  Add/1 -> Out1/1
  Interval Test1/1 -> Switch1/2
  Switch/1 -> Add/1
  Interval Test/1 -> Switch/2
  Clock/1 -> Gain/1

== system Microgrid_W/House 5 W3/Lamp 2/D3 ==
  Add : Sum
  Clock : Clock
  Constant : Constant
  Constant1 : Constant  Value=0
  Gain : Gain  Gain=t
  Interval Test : simulink/Logic and Bit Operations/Interval Test  IntervalClosedRight=on  uplimit=L2_Off_1+86400*2  IntervalClosedLeft=on  lowlimit=L2_On_1+86400*2  OutDataTypeStr=boolean
  Interval Test1 : simulink/Logic and Bit Operations/Interval Test  IntervalClosedRight=on  uplimit=L2_Off_2+86400*2  IntervalClosedLeft=on  lowlimit=L2_On_2+86400*2  OutDataTypeStr=boolean
  Switch : Switch  Criteria=u2 > Threshold  Threshold=0.5
  Switch1 : Switch  Criteria=u2 > Threshold  Threshold=0.5
  Out1 : Outport  VectorParamsAs1DForOutWhenUnconnected=off
  wires:
  Interval Test/1 -> Switch/2
  Switch/1 -> Add/1
  Interval Test1/1 -> Switch1/2
  Add/1 -> Out1/1
  Constant1/1 -> Switch/3, Switch1/3
  Constant/1 -> Switch/1, Switch1/1
  Switch1/1 -> Add/2
  Gain/1 -> Interval Test1/1, Interval Test/1
  Clock/1 -> Gain/1

== system Microgrid_W/House 5 W3/Lamp 2/D4 ==
  Add : Sum
  Clock : Clock
  Constant : Constant
  Constant1 : Constant  Value=0
  Gain : Gain  Gain=t
  Interval Test : simulink/Logic and Bit Operations/Interval Test  IntervalClosedRight=on  uplimit=L2_Off_1+86400*3  IntervalClosedLeft=on  lowlimit=L2_On_1+86400*3  OutDataTypeStr=boolean
  Interval Test1 : simulink/Logic and Bit Operations/Interval Test  IntervalClosedRight=on  uplimit=L2_Off_2+86400*3  IntervalClosedLeft=on  lowlimit=L2_On_2+86400*3  OutDataTypeStr=boolean
  Switch : Switch  Criteria=u2 > Threshold  Threshold=0.5
  Switch1 : Switch  Criteria=u2 > Threshold  Threshold=0.5
  Out1 : Outport  VectorParamsAs1DForOutWhenUnconnected=off
  wires:
  Gain/1 -> Interval Test/1, Interval Test1/1
  Switch1/1 -> Add/2
  Constant/1 -> Switch1/1, Switch/1
  Constant1/1 -> Switch1/3, Switch/3
  Add/1 -> Out1/1
  Interval Test1/1 -> Switch1/2
  Switch/1 -> Add/1
  Interval Test/1 -> Switch/2
  Clock/1 -> Gain/1

== system Microgrid_W/House 5 W3/Lamp 2/D5 ==
  Add : Sum
  Clock : Clock
  Constant : Constant
  Constant1 : Constant  Value=0
  Gain : Gain  Gain=t
  Interval Test : simulink/Logic and Bit Operations/Interval Test  IntervalClosedRight=on  uplimit=L2_Off_1+86400*4  IntervalClosedLeft=on  lowlimit=L2_On_1+86400*4  OutDataTypeStr=boolean
  Interval Test1 : simulink/Logic and Bit Operations/Interval Test  IntervalClosedRight=on  uplimit=L2_Off_2+86400*4  IntervalClosedLeft=on  lowlimit=L2_On_2+86400*4  OutDataTypeStr=boolean
  Switch : Switch  Criteria=u2 > Threshold  Threshold=0.5
  Switch1 : Switch  Criteria=u2 > Threshold  Threshold=0.5
  Out1 : Outport  VectorParamsAs1DForOutWhenUnconnected=off
  wires:
  Interval Test/1 -> Switch/2
  Switch/1 -> Add/1
  Interval Test1/1 -> Switch1/2
  Add/1 -> Out1/1
  Constant1/1 -> Switch/3, Switch1/3
  Constant/1 -> Switch/1, Switch1/1
  Switch1/1 -> Add/2
  Gain/1 -> Interval Test1/1, Interval Test/1
  Clock/1 -> Gain/1

== system Microgrid_W/House 5 W3/Lamp 2/D6 ==
  Add : Sum
  Clock : Clock
  Constant : Constant
  Constant1 : Constant  Value=0
  Gain : Gain  Gain=t
  Interval Test : simulink/Logic and Bit Operations/Interval Test  IntervalClosedRight=on  uplimit=L2_Off_1+86400*5  IntervalClosedLeft=on  lowlimit=L2_On_1+86400*5  OutDataTypeStr=boolean
  Interval Test1 : simulink/Logic and Bit Operations/Interval Test  IntervalClosedRight=on  uplimit=L2_Off_2+86400*5  IntervalClosedLeft=on  lowlimit=L2_On_2+86400*5  OutDataTypeStr=boolean
  Switch : Switch  Criteria=u2 > Threshold  Threshold=0.5
  Switch1 : Switch  Criteria=u2 > Threshold  Threshold=0.5
  Out1 : Outport  VectorParamsAs1DForOutWhenUnconnected=off
  wires:
  Gain/1 -> Interval Test/1, Interval Test1/1
  Switch1/1 -> Add/2
  Constant/1 -> Switch1/1, Switch/1
  Constant1/1 -> Switch1/3, Switch/3
  Add/1 -> Out1/1
  Interval Test1/1 -> Switch1/2
  Switch/1 -> Add/1
  Interval Test/1 -> Switch/2
  Clock/1 -> Gain/1

== system Microgrid_W/House 5 W3/Lamp 2/D7 ==
  Add : Sum
  Clock : Clock
  Constant : Constant
  Constant1 : Constant  Value=0
  Gain : Gain  Gain=t
  Interval Test : simulink/Logic and Bit Operations/Interval Test  IntervalClosedRight=on  uplimit=L2_Off_1+86400*6  IntervalClosedLeft=on  lowlimit=L2_On_1+86400*6  OutDataTypeStr=boolean
  Interval Test1 : simulink/Logic and Bit Operations/Interval Test  IntervalClosedRight=on  uplimit=L2_Off_2+86400*6  IntervalClosedLeft=on  lowlimit=L2_On_2+86400*6  OutDataTypeStr=boolean
  Switch : Switch  Criteria=u2 > Threshold  Threshold=0.5
  Switch1 : Switch  Criteria=u2 > Threshold  Threshold=0.5
  Out1 : Outport  VectorParamsAs1DForOutWhenUnconnected=off
  wires:
  Interval Test/1 -> Switch/2
  Switch/1 -> Add/1
  Interval Test1/1 -> Switch1/2
  Add/1 -> Out1/1
  Constant1/1 -> Switch/3, Switch1/3
  Constant/1 -> Switch/1, Switch1/1
  Switch1/1 -> Add/2
  Gain/1 -> Interval Test1/1, Interval Test/1
  Clock/1 -> Gain/1

== system Microgrid_W/House 5 W3/Lamp 3/D1 ==
  Add : Sum
  Clock : Clock
  Constant : Constant
  Constant1 : Constant  Value=0
  Gain : Gain  Gain=t
  Interval Test : simulink/Logic and Bit Operations/Interval Test  IntervalClosedRight=on  uplimit=L3_Off_1  IntervalClosedLeft=on  lowlimit=L3_On_1  OutDataTypeStr=boolean
  Interval Test1 : simulink/Logic and Bit Operations/Interval Test  IntervalClosedRight=on  uplimit=L3_Off_2  IntervalClosedLeft=on  lowlimit=L3_On_2  OutDataTypeStr=boolean
  Switch : Switch  Criteria=u2 > Threshold  Threshold=0.5
  Switch1 : Switch  Criteria=u2 > Threshold  Threshold=0.5
  Out1 : Outport  VectorParamsAs1DForOutWhenUnconnected=off
  wires:
  Gain/1 -> Interval Test/1, Interval Test1/1
  Switch1/1 -> Add/2
  Constant/1 -> Switch1/1, Switch/1
  Constant1/1 -> Switch1/3, Switch/3
  Add/1 -> Out1/1
  Interval Test1/1 -> Switch1/2
  Switch/1 -> Add/1
  Interval Test/1 -> Switch/2
  Clock/1 -> Gain/1

== system Microgrid_W/House 5 W3/Lamp 3/D2 ==
  Add : Sum
  Clock : Clock
  Constant : Constant
  Constant1 : Constant  Value=0
  Gain : Gain  Gain=t
  Interval Test : simulink/Logic and Bit Operations/Interval Test  IntervalClosedRight=on  uplimit=L3_Off_1+86400  IntervalClosedLeft=on  lowlimit=L3_On_1+86400  OutDataTypeStr=boolean
  Interval Test1 : simulink/Logic and Bit Operations/Interval Test  IntervalClosedRight=on  uplimit=L3_Off_2+86400  IntervalClosedLeft=on  lowlimit=L3_On_2+86400  OutDataTypeStr=boolean
  Switch : Switch  Criteria=u2 > Threshold  Threshold=0.5
  Switch1 : Switch  Criteria=u2 > Threshold  Threshold=0.5
  Out1 : Outport  VectorParamsAs1DForOutWhenUnconnected=off
  wires:
  Interval Test/1 -> Switch/2
  Switch/1 -> Add/1
  Interval Test1/1 -> Switch1/2
  Add/1 -> Out1/1
  Constant1/1 -> Switch/3, Switch1/3
  Constant/1 -> Switch/1, Switch1/1
  Switch1/1 -> Add/2
  Gain/1 -> Interval Test1/1, Interval Test/1
  Clock/1 -> Gain/1

== system Microgrid_W/House 5 W3/Lamp 3/D3 ==
  Add : Sum
  Clock : Clock
  Constant : Constant
  Constant1 : Constant  Value=0
  Gain : Gain  Gain=t
  Interval Test : simulink/Logic and Bit Operations/Interval Test  IntervalClosedRight=on  uplimit=L3_Off_1+86400*2  IntervalClosedLeft=on  lowlimit=L3_On_1+86400*2  OutDataTypeStr=boolean
  Interval Test1 : simulink/Logic and Bit Operations/Interval Test  IntervalClosedRight=on  uplimit=L3_Off_2+86400*2  IntervalClosedLeft=on  lowlimit=L3_On_2+86400*2  OutDataTypeStr=boolean
  Switch : Switch  Criteria=u2 > Threshold  Threshold=0.5
  Switch1 : Switch  Criteria=u2 > Threshold  Threshold=0.5
  Out1 : Outport  VectorParamsAs1DForOutWhenUnconnected=off
  wires:
  Gain/1 -> Interval Test/1, Interval Test1/1
  Switch1/1 -> Add/2
  Constant/1 -> Switch1/1, Switch/1
  Constant1/1 -> Switch1/3, Switch/3
  Add/1 -> Out1/1
  Interval Test1/1 -> Switch1/2
  Switch/1 -> Add/1
  Interval Test/1 -> Switch/2
  Clock/1 -> Gain/1

== system Microgrid_W/House 5 W3/Lamp 3/D4 ==
  Add : Sum
  Clock : Clock
  Constant : Constant
  Constant1 : Constant  Value=0
  Gain : Gain  Gain=t
  Interval Test : simulink/Logic and Bit Operations/Interval Test  IntervalClosedRight=on  uplimit=L3_Off_1+86400*3  IntervalClosedLeft=on  lowlimit=L3_On_1+86400*3  OutDataTypeStr=boolean
  Interval Test1 : simulink/Logic and Bit Operations/Interval Test  IntervalClosedRight=on  uplimit=L3_Off_2+86400*3  IntervalClosedLeft=on  lowlimit=L3_On_2+86400*3  OutDataTypeStr=boolean
  Switch : Switch  Criteria=u2 > Threshold  Threshold=0.5
  Switch1 : Switch  Criteria=u2 > Threshold  Threshold=0.5
  Out1 : Outport  VectorParamsAs1DForOutWhenUnconnected=off
  wires:
  Interval Test/1 -> Switch/2
  Switch/1 -> Add/1
  Interval Test1/1 -> Switch1/2
  Add/1 -> Out1/1
  Constant1/1 -> Switch/3, Switch1/3
  Constant/1 -> Switch/1, Switch1/1
  Switch1/1 -> Add/2
  Gain/1 -> Interval Test1/1, Interval Test/1
  Clock/1 -> Gain/1

== system Microgrid_W/House 5 W3/Lamp 3/D5 ==
  Add : Sum
  Clock : Clock
  Constant : Constant
  Constant1 : Constant  Value=0
  Gain : Gain  Gain=t
  Interval Test : simulink/Logic and Bit Operations/Interval Test  IntervalClosedRight=on  uplimit=L3_Off_1+86400*4  IntervalClosedLeft=on  lowlimit=L3_On_1+86400*4  OutDataTypeStr=boolean
  Interval Test1 : simulink/Logic and Bit Operations/Interval Test  IntervalClosedRight=on  uplimit=L3_Off_2+86400*4  IntervalClosedLeft=on  lowlimit=L3_On_2+86400*4  OutDataTypeStr=boolean
  Switch : Switch  Criteria=u2 > Threshold  Threshold=0.5
  Switch1 : Switch  Criteria=u2 > Threshold  Threshold=0.5
  Out1 : Outport  VectorParamsAs1DForOutWhenUnconnected=off
  wires:
  Gain/1 -> Interval Test/1, Interval Test1/1
  Switch1/1 -> Add/2
  Constant/1 -> Switch1/1, Switch/1
  Constant1/1 -> Switch1/3, Switch/3
  Add/1 -> Out1/1
  Interval Test1/1 -> Switch1/2
  Switch/1 -> Add/1
  Interval Test/1 -> Switch/2
  Clock/1 -> Gain/1

== system Microgrid_W/House 5 W3/Lamp 3/D6 ==
  Add : Sum
  Clock : Clock
  Constant : Constant
  Constant1 : Constant  Value=0
  Gain : Gain  Gain=t
  Interval Test : simulink/Logic and Bit Operations/Interval Test  IntervalClosedRight=on  uplimit=L3_Off_1+86400*5  IntervalClosedLeft=on  lowlimit=L3_On_1+86400*5  OutDataTypeStr=boolean
  Interval Test1 : simulink/Logic and Bit Operations/Interval Test  IntervalClosedRight=on  uplimit=L3_Off_2+86400*5  IntervalClosedLeft=on  lowlimit=L3_On_2+86400*5  OutDataTypeStr=boolean
  Switch : Switch  Criteria=u2 > Threshold  Threshold=0.5
  Switch1 : Switch  Criteria=u2 > Threshold  Threshold=0.5
  Out1 : Outport  VectorParamsAs1DForOutWhenUnconnected=off
  wires:
  Interval Test/1 -> Switch/2
  Switch/1 -> Add/1
  Interval Test1/1 -> Switch1/2
  Add/1 -> Out1/1
  Constant1/1 -> Switch/3, Switch1/3
  Constant/1 -> Switch/1, Switch1/1
  Switch1/1 -> Add/2
  Gain/1 -> Interval Test1/1, Interval Test/1
  Clock/1 -> Gain/1

== system Microgrid_W/House 5 W3/Lamp 3/D7 ==
  Add : Sum
  Clock : Clock
  Constant : Constant
  Constant1 : Constant  Value=0
  Gain : Gain  Gain=t
  Interval Test : simulink/Logic and Bit Operations/Interval Test  IntervalClosedRight=on  uplimit=L3_Off_1+86400*6  IntervalClosedLeft=on  lowlimit=L3_On_1+86400*6  OutDataTypeStr=boolean
  Interval Test1 : simulink/Logic and Bit Operations/Interval Test  IntervalClosedRight=on  uplimit=L3_Off_2+86400*6  IntervalClosedLeft=on  lowlimit=L3_On_2+86400*6  OutDataTypeStr=boolean
  Switch : Switch  Criteria=u2 > Threshold  Threshold=0.5
  Switch1 : Switch  Criteria=u2 > Threshold  Threshold=0.5
  Out1 : Outport  VectorParamsAs1DForOutWhenUnconnected=off
  wires:
  Gain/1 -> Interval Test/1, Interval Test1/1
  Switch1/1 -> Add/2
  Constant/1 -> Switch1/1, Switch/1
  Constant1/1 -> Switch1/3, Switch/3
  Add/1 -> Out1/1
  Interval Test1/1 -> Switch1/2
  Switch/1 -> Add/1
  Interval Test/1 -> Switch/2
  Clock/1 -> Gain/1

== system Microgrid_W/House 5 W3/Laptop_Charger/D1 ==
  Add : Sum
  Clock : Clock
  Constant : Constant
  Constant1 : Constant  Value=0
  Gain : Gain  Gain=t
  Interval Test : simulink/Logic and Bit Operations/Interval Test  IntervalClosedRight=on  uplimit=Laptop_C_2_Off_a  IntervalClosedLeft=on  lowlimit=Laptop_C_2_On_a  OutDataTypeStr=boolean
  Interval Test1 : simulink/Logic and Bit Operations/Interval Test  IntervalClosedRight=on  uplimit=Laptop_C_2_Off_b  IntervalClosedLeft=on  lowlimit=Laptop_C_2_On_b  OutDataTypeStr=boolean
  Switch : Switch  Criteria=u2 > Threshold  Threshold=0.5
  Switch1 : Switch  Criteria=u2 > Threshold  Threshold=0.5
  Out1 : Outport  VectorParamsAs1DForOutWhenUnconnected=off
  wires:
  Gain/1 -> Interval Test/1, Interval Test1/1
  Switch1/1 -> Add/2
  Constant/1 -> Switch1/1, Switch/1
  Constant1/1 -> Switch1/3, Switch/3
  Add/1 -> Out1/1
  Interval Test1/1 -> Switch1/2
  Switch/1 -> Add/1
  Interval Test/1 -> Switch/2
  Clock/1 -> Gain/1

== system Microgrid_W/House 5 W3/Laptop_Charger/D10 ==
  Clock : Clock
  Constant : Constant
  Constant1 : Constant  Value=0
  Gain : Gain  Gain=t
  Interval Test : simulink/Logic and Bit Operations/Interval Test  IntervalClosedRight=on  uplimit=Laptop_C_1_Off_a+86400*2  IntervalClosedLeft=on  lowlimit=Laptop_C_1_On_a+86400*2  OutDataTypeStr=boolean
  Switch : Switch  Criteria=u2 > Threshold  Threshold=0.5
  Out1 : Outport  VectorParamsAs1DForOutWhenUnconnected=off
  wires:
  Interval Test/1 -> Switch/2
  Switch/1 -> Out1/1
  Constant1/1 -> Switch/3
  Constant/1 -> Switch/1
  Gain/1 -> Interval Test/1
  Clock/1 -> Gain/1

== system Microgrid_W/House 5 W3/Laptop_Charger/D11 ==
  Clock : Clock
  Constant : Constant
  Constant1 : Constant  Value=0
  Gain : Gain  Gain=t
  Interval Test : simulink/Logic and Bit Operations/Interval Test  IntervalClosedRight=on  uplimit=Laptop_C_1_Off_a+86400*3  IntervalClosedLeft=on  lowlimit=Laptop_C_1_On_a+86400*3  OutDataTypeStr=boolean
  Switch : Switch  Criteria=u2 > Threshold  Threshold=0.5
  Out1 : Outport  VectorParamsAs1DForOutWhenUnconnected=off
  wires:
  Gain/1 -> Interval Test/1
  Constant/1 -> Switch/1
  Constant1/1 -> Switch/3
  Switch/1 -> Out1/1
  Interval Test/1 -> Switch/2
  Clock/1 -> Gain/1
